simulink model "problem_1"  (R2020b)
settings: Solver=VariableStepAuto  StartTime=0.0  StopTime=10.0  RelTol=1e-3
model workspace (MAT data in the model file):
  b = Simulink.Parameter
  b.Value = 50
  b.DataType = 'auto'
  b.Dimensions = [1 1]
  k1 = Simulink.Parameter
  k1.Value = 50
  k1.DataType = 'auto'
  k1.Dimensions = [1 1]
  k12 = Simulink.Parameter
  k12.Value = 10
  k12.DataType = 'auto'
  k12.Dimensions = [1 1]
  m1 = Simulink.Parameter
  m1.Value = 100
  m1.DataType = 'auto'
  m1.Dimensions = [1 1]
  m2 = Simulink.Parameter
  m2.Value = 100
  m2.DataType = 'auto'
  m2.Dimensions = [1 1]
settings Model: Creator=k.Raviteja  LastModifiedBy=k.Raviteja

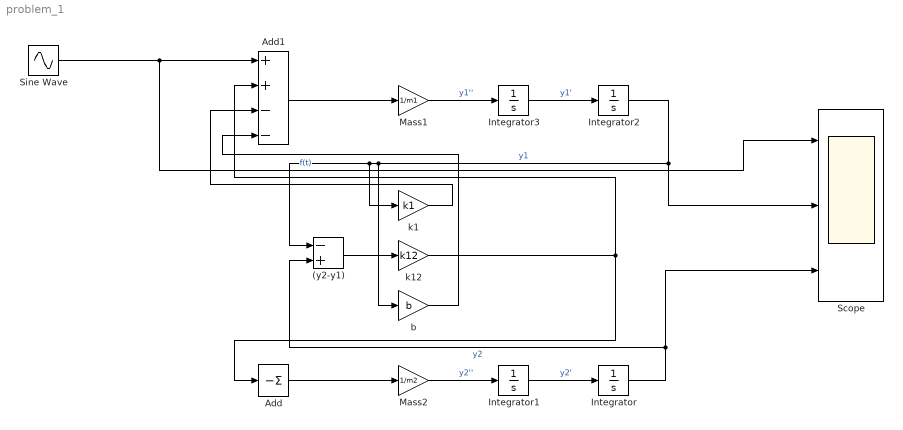
== system problem_1 ==
  (y2-y1) : Sum  Inputs=-+
  Add : Sum  Inputs=-
  Add1 : Sum  Inputs=++--
  Integrator{,1..3} (4 alike) : Integrator
  Mass1 : Gain  Gain=1/m1
  Mass2 : Gain  Gain=1/m2
  Scope : Scope  NumInputPorts=3
  Sine Wave : Sin  Amplitude=2  Frequency=10/(2*pi)  SampleTime=0
  b : Gain  Gain=b
  k1 : Gain  Gain=k1
  k12 : Gain  Gain=k12
  wires:
  Integrator1/1 -> Integrator/1  "y2'"
  Integrator3/1 -> Integrator2/1  "y1'"
  Mass1/1 -> Integrator3/1  "y1''"
  Mass2/1 -> Integrator1/1  "y2''"
  Integrator2/1 -> Scope/2, b/1, k1/1, (y2-y1)/1  "y1"
  Integrator/1 -> Scope/3, (y2-y1)/2  "y2"
  Add/1 -> Mass2/1
  Add1/1 -> Mass1/1
  (y2-y1)/1 -> k12/1
  k12/1 -> Add1/2, Add/1
  k1/1 -> Add1/3
  b/1 -> Add1/4
  Sine Wave/1 -> Scope/1, Add1/1  "f(t)"
